simulink model "laba1"  (Simulink 7.2)
settings: Solver=ode45  StartTime=0.0  StopTime=10.0  RelTol=1e-3
settings Model: Creator=imalov  LastModifiedBy=imalov

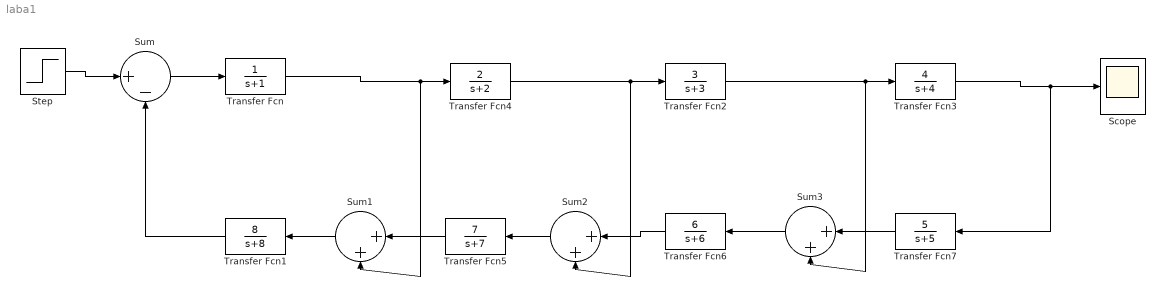
== system laba1 ==
  Scope : Scope
  Step : Step  SampleTime=0
  Sum : Sum  Inputs=|+-  OutDataType=sfix(16)  OutScaling=2^0
  Sum1 : Sum  Orientation=left  Inputs=|++  OutDataType=sfix(16)  OutScaling=2^0
  Sum2 : Sum  Orientation=left  Inputs=|++  OutDataType=sfix(16)  OutScaling=2^0
  Sum3 : Sum  Orientation=left  Inputs=|++  OutDataType=sfix(16)  OutScaling=2^0
  Transfer Fcn : TransferFcn  Denominator=[1 1]
  Transfer Fcn1 : TransferFcn  Orientation=left  Numerator=[8]  Denominator=[1 8]
  Transfer Fcn2 : TransferFcn  Numerator=[3]  Denominator=[1 3]
  Transfer Fcn3 : TransferFcn  Numerator=[4]  Denominator=[1 4]
  Transfer Fcn4 : TransferFcn  Numerator=[2]  Denominator=[1 2]
  Transfer Fcn5 : TransferFcn  Orientation=left  Numerator=[7]  Denominator=[1 7]
  Transfer Fcn6 : TransferFcn  Orientation=left  Numerator=[6]  Denominator=[1 6]
  Transfer Fcn7 : TransferFcn  Orientation=left  Numerator=[5]  Denominator=[1 5]
  wires:
  Step/1 -> Sum/1
  Transfer Fcn/1 -> Transfer Fcn4/1, Sum1/2
  Transfer Fcn4/1 -> Transfer Fcn2/1, Sum2/2
  Transfer Fcn2/1 -> Transfer Fcn3/1, Sum3/2
  Transfer Fcn3/1 -> Scope/1, Transfer Fcn7/1
  Transfer Fcn7/1 -> Sum3/1
  Sum3/1 -> Transfer Fcn6/1
  Transfer Fcn6/1 -> Sum2/1
  Sum2/1 -> Transfer Fcn5/1
  Transfer Fcn5/1 -> Sum1/1
  Sum1/1 -> Transfer Fcn1/1
  Transfer Fcn1/1 -> Sum/2
  Sum/1 -> Transfer Fcn/1
